simulink model "positivebuckboostFinalA"  (Simulink 7.8)
settings: Solver=ode45  StartTime=0.0  StopTime=1  RelTol=1e-3
libraries: powerlib x15, simulink x5, powerlib_extras x1
settings Model: Creator=mictu  LastModifiedBy=mictu
settings DebuggingCC: FcnCallInpInsideContextMsg=Use local settings

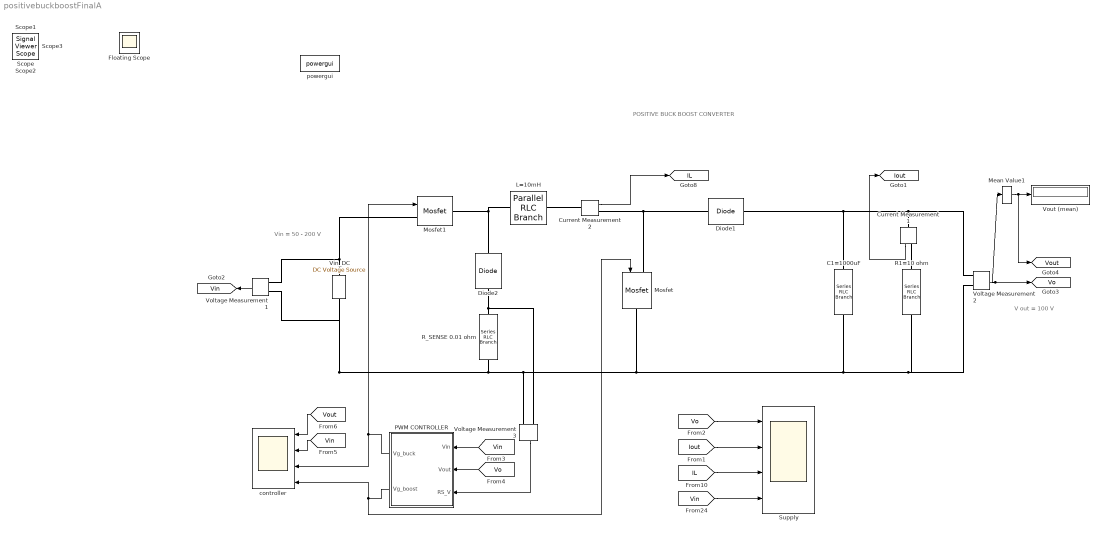
== system positivebuckboostFinalA ==
  note: Vin = 50 - 200 V
  note: V out = 100 V
  note: POSITIVE BUCK BOOST CONVERTER
  C1=1000uF : powerlib/Elements/Series RLC Branch  LConnTagsString=__new0  RConnTagsString=__new0  BranchType=C  Resistance=100e-3  Inductance=1e-3  SetiL0=off  InitialCurrent=0  Capacitance=100e-6  Setx0=off  InitialVoltage=0  Measurements=None
  Current Measurement1 : powerlib/Measurements/Current Measurement  PhasorSimulation=off  OutputType=Complex  PSBequivalent=0
  Current Measurement2 : powerlib/Measurements/Current Measurement  PhasorSimulation=off  OutputType=Complex  PSBequivalent=0
  Diode1 : powerlib/Power Electronics/Diode  Ron=0.001  Lon=0  Vf=0.8  IC=0  UseSnubber=off  Rs=500  Cs=250e-9  Measurements=off
  Diode2 : powerlib/Power Electronics/Diode  Ron=0.001  Lon=0  Vf=0.8  IC=0  UseSnubber=off  Rs=500  Cs=250e-9  Measurements=off
  L=10mH : powerlib/Elements/Parallel RLC Branch  LConnTagsString=a  RConnTagsString=__new0  BranchType=L  Resistance=1.0  Inductance=10e-3  SetiL0=off  InitialCurrent=0  Capacitance=1.0  Setx0=off  InitialVoltage=0  Measurements=None
  Mean Value1 : powerlib_extras/Measurements/Mean Value  Period=10e-3
  Mosfet : powerlib/Power Electronics/Mosfet  Ron=0.001  Lon=0  Rd=0.001  Vfd=0  IC=0  Rs=10  Cs=0.047e-6  Measurements=off
  Mosfet1 : powerlib/Power Electronics/Mosfet  Ron=0.001  Lon=0  Rd=0.001  Vfd=0  IC=0  Rs=10  Cs=0.047e-6  Measurements=off
  PWM CONTROLLER : Subsystem
  R1=10 ohm : powerlib/Elements/Series RLC Branch  LConnTagsString=__new0  RConnTagsString=__new0  BranchType=R  Resistance=10  Inductance=1e-3  SetiL0=off  InitialCurrent=0  Capacitance=100e-6  Setx0=off  InitialVoltage=0  Measurements=None
  R_SENSE 0.01 ohm : powerlib/Elements/Series RLC Branch  LConnTagsString=__new0  RConnTagsString=__new0  BranchType=R  Resistance=0.01  Inductance=1e-3  SetiL0=off  InitialCurrent=0  Capacitance=100e-6  Setx0=off  InitialVoltage=0  Measurements=None
  Supply : Scope  NumInputPorts=4
      settings: YMin=0~42750~0~-5  YMax=1~47250~14~60  MaxDataPoints=10000
  Vin_DC : powerlib/Electrical Sources/DC Voltage Source  Amplitude=100  Measurements=None
  Voltage Measurement1 : powerlib/Measurements/Voltage Measurement  PhasorSimulation=off  OutputType=Complex  PSBequivalent=0
  Voltage Measurement2 : powerlib/Measurements/Voltage Measurement  PhasorSimulation=off  OutputType=Complex  PSBequivalent=0
  Voltage Measurement3 : powerlib/Measurements/Voltage Measurement  PhasorSimulation=off  OutputType=Complex  PSBequivalent=0
  Vout (mean) : Display
      settings: SampleTime=1e-3
  controller : Scope  NumInputPorts=4
      settings: TimeRange=0.0005234781529580984  YMin=90~195~1~-1  YMax=110~205~1~2  MaxDataPoints=10000
  powergui : powerlib/powergui  SimulationMode=Discrete  SolverType=Tustin  SampleTime=1e-6  frequency=60  SPID=off  DisableSnubberDevices=off  DisableRonSwitches=off  DisableVfSwitches=off  SwTol=0  Interpol=off  DisplayEquations=off  FunctionMessages=off  frequencyindice=0  Pbase=100e6  ErrMax=1e-4  Iterations=50  UnitsV=kV  UnitsW=MW  echomessages=off  HookPort=off  EnableUseOfTLC=off  x0status=blocks  RestoreLinks=warning  ResistiveCurrentMeasurement=off  Frange=[0:2:500]  Ylog=off  Xlog=on  ShowGrid=off  save=off  variable=ZData  ZoomFFT=on  StartTime=0.0  cycles=1  DisplayStyle=1  fundamental=60  FreqAxis=off  MaxFrequency=1000  frequencyindicesteady=1  RmsSteady=1  display=off  Ts=0  methode=off
  Floating Scope : Scope
      settings: Floating=on  SaveName=ScopeData2
  Scope : SignalViewerScope  IOType=viewer  ZoomMode=xonly  RefreshTime=0.035000
  Scope1 : SignalViewerScope  IOType=viewer  RefreshTime=0.035000
  Scope2 : SignalViewerScope  IOType=viewer  ZoomMode=xonly  RefreshTime=0.035000
      settings: SaveName=ScopeData2
  Scope3 : SignalViewerScope  IOType=viewer  ZoomMode=xonly  RefreshTime=0.035000
      settings: SaveName=ScopeData3
  tag scope: IL=global, Iout=global, Vin=global, Vo=global, Vout=global
  wires:
  Voltage Measurement1/1 -> [Vin]
  Current Measurement2/1 -> [IL]
  Voltage Measurement2/1 -> [Vo], Mean Value1/1
  [Vo] -> Supply/1
  [Vin] -> Supply/4
  [IL] -> Supply/3
  Current Measurement1/1 -> [Iout]
  [Iout] -> Supply/2
  [Vin] -> PWM CONTROLLER/1(Vin)
  [Vo] -> PWM CONTROLLER/2(Vout)
  PWM CONTROLLER/1(Vg_buck) -> Mosfet1/1, controller/3
  Mean Value1/1 -> Vout (mean)/1, [Vout]
  PWM CONTROLLER/2(Vg_boost) -> Mosfet/1, controller/4
  Voltage Measurement3/1 -> PWM CONTROLLER/3(RS_V)
  [Vout] -> controller/1
  [Vin] -> controller/2
  connections:
  Diode2/RConn1 -- L=10mH/LConn1 -- Mosfet1/RConn1
  Mosfet/LConn1 -- Diode1/LConn1 -- Current Measurement2/RConn1
  R1=10 ohm/RConn1 -- Voltage Measurement2/LConn2 -- C1=1000uF/RConn1 -- Mosfet/RConn1 -- Vin_DC/LConn1 -- Voltage Measurement1/LConn2 -- R_SENSE 0.01 ohm/RConn1 -- Voltage Measurement3/LConn1
  Mosfet1/LConn1 -- Vin_DC/RConn1 -- Voltage Measurement1/LConn1
  Voltage Measurement2/LConn1 -- Diode1/RConn1 -- C1=1000uF/LConn1 -- Current Measurement1/LConn1
  Current Measurement2/LConn1 -- L=10mH/RConn1
  Current Measurement1/RConn1 -- R1=10 ohm/LConn1
  Diode2/LConn1 -- R_SENSE 0.01 ohm/LConn1 -- Voltage Measurement3/LConn2

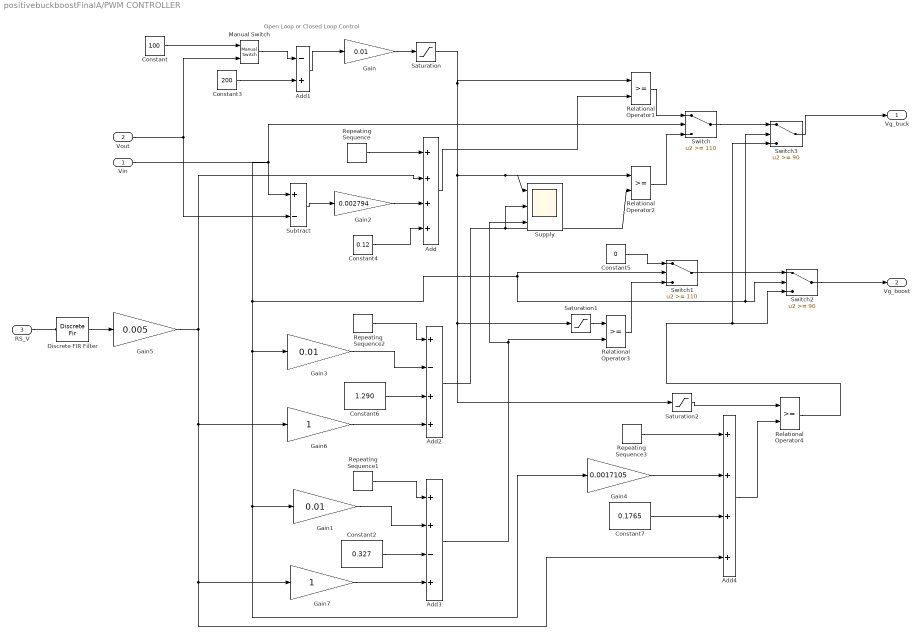
== system positivebuckboostFinalA/PWM CONTROLLER ==
  note: Open Loop
      | or
      |  Closed Loop
      | Control
  Vin : Inport
  Vout : Inport  Port=2
  RS_V : Inport  Port=3
  Add : Sum  Inputs=++++
  Add1 : Sum  Inputs=-+
  Add2 : Sum  Inputs=+-++
  Add3 : Sum  Inputs=++-+
  Add4 : Sum  Inputs=++++
  Constant : Constant  Value=100
  Constant2 : Constant  Value=0.327
  Constant3 : Constant  Value=200
  Constant4 : Constant  Value=0.12
  Constant5 : Constant  Value=0
  Constant6 : Constant  Value=1.290
  Constant7 : Constant  Value=0.1765
  Discrete FIR Filter : DiscreteFir  SampleTime=1e-3  AccumDataTypeStr=Inherit: Same as product output
  Gain : Gain  Gain=0.01
  Gain1 : Gain  Gain=0.01
  Gain2 : Gain  Gain=0.002794
  Gain3 : Gain  Gain=0.01
  Gain4 : Gain  Gain=0.0017105
  Gain5 : Gain  Gain=0.005
  Gain6 : Gain
  Gain7 : Gain
  Manual Switch : simulink/Signal Routing/Manual Switch  sw=0  action=0  varsize=off
  Relational Operator{1..4} (4 alike) : RelationalOperator  InputSameDT=on
  Repeating Sequence : simulink/Sources/Repeating Sequence  rep_seq_t=[0 1/10e3]  rep_seq_y=[0.25 0.92]
  Repeating Sequence1 : simulink/Sources/Repeating Sequence  rep_seq_t=[0 1/10e3]  rep_seq_y=[0.2 0.61667]
  Repeating Sequence2 : simulink/Sources/Repeating Sequence  rep_seq_t=[0 1/10e3]  rep_seq_y=[0.2 0.9143]
  Repeating Sequence3 : simulink/Sources/Repeating Sequence  rep_seq_t=[0 1/10e3]  rep_seq_y=[0.402 0.902]
  Saturation : Saturate  UpperLimit=0.995  LowerLimit=0
  Saturation1 : Saturate  UpperLimit=0.995  LowerLimit=0.994
  Saturation2 : Saturate  UpperLimit=0.995  LowerLimit=0.9949
  Subtract : Sum  Inputs=+-
  Supply : Scope  NumInputPorts=3
      settings: YMin=0~0.1~0.4  YMax=1~1.35~1.5  SaveName=ScopeData3  MaxDataPoints=10000
  Switch : Switch  Threshold=110
  Switch1 : Switch  Threshold=110
  Switch2 : Switch  Threshold=90
  Switch3 : Switch  Threshold=90
  Vg_buck : Outport
  Vg_boost : Outport  Port=2
  wires:
  Constant/1 -> Manual Switch/1
  Gain/1 -> Saturation/1
  Repeating Sequence/1 -> Add/1
  Vin/1 -> Subtract/1, Switch/2, Gain3/1, Gain1/1, Gain4/1, Switch1/2, Switch2/2, Switch3/2
  Vout/1 -> Subtract/2, Manual Switch/2
  Subtract/1 -> Gain2/1
  Add1/1 -> Gain/1
  Constant3/1 -> Add1/2
  Manual Switch/1 -> Add1/1
  ? -> ?
  Constant6/1 -> Add2/3
  ? -> ?
  Add/1 -> Relational Operator1/2
  Relational Operator1/1 -> Switch/1
  Relational Operator2/1 -> Switch/3
  Saturation/1 -> Relational Operator1/1, Saturation1/1, Saturation2/1, Relational Operator2/1, Supply/1
  Add2/1 -> Relational Operator2/2, Supply/2
  Repeating Sequence1/1 -> Add3/1
  Constant2/1 -> Add3/3
  Gain1/1 -> Add3/2
  Repeating Sequence2/1 -> Add2/1
  Gain3/1 -> Add2/2
  Add3/1 -> Relational Operator3/2, Supply/3
  Relational Operator3/1 -> Switch1/3
  Constant5/1 -> Switch1/1
  Saturation1/1 -> Relational Operator3/1
  Repeating Sequence3/1 -> Add4/1
  Gain4/1 -> Add4/2
  Constant7/1 -> Add4/3
  Add4/1 -> Relational Operator4/2
  Relational Operator4/1 -> Switch2/3, Switch3/3
  Switch1/1 -> Switch2/1
  Switch2/1 -> Vg_boost/1
  Switch/1 -> Switch3/1
  Switch3/1 -> Vg_buck/1
  Saturation2/1 -> Relational Operator4/1
  RS_V/1 -> Discrete FIR Filter/1
  Discrete FIR Filter/1 -> Gain5/1
  Gain5/1 -> Add4/4, Gain7/1, Gain6/1, Add/2
  Gain6/1 -> Add2/4
  Gain7/1 -> Add3/4
  Gain2/1 -> Add/3
  Constant4/1 -> Add/4
